simulink model "Integrate_and_fire_STDP"  (R2019b)
settings: Solver=VariableStepAuto  StartTime=0.0  StopTime=1  RelTol=1e-3
libraries: NeuroModelerLibrary x4
settings Model: Creator=Oleg  LastModifiedBy=Bakhshiev
settings DataIOCC: ReturnWorkspaceOutputs=off
settings DebuggingCC: ArithmeticOperatorsInVariantConditions=warning
settings SFSimCC: SimUseLocalCustomCode=off  CustomCodeUndefinedFunction=UseInterfaceOnly
settings RTWCC: RTWUseLocalCustomCode=off
settings CodeAppCC: StateflowObjectComments=on

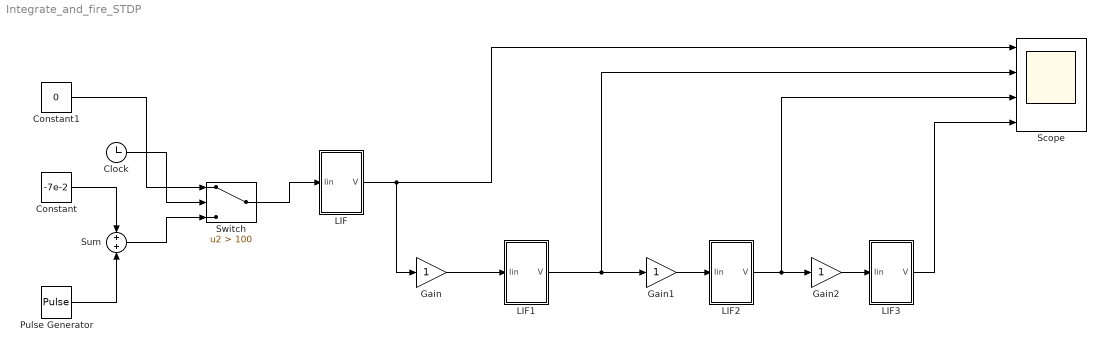
== system Integrate_and_fire_STDP ==
  Clock : Clock
  Constant : Constant  Value=-7e-2
  Constant1 : Constant  Value=0
  Gain : Gain
  Gain1 : Gain
  Gain2 : Gain
  LIF : Subsystem  mask{gL=3e-8, VL=-7e-2, C=1e-11, VT=-5e-2, Vreset=3e-2}
      mask prompts: gL "membraneConductivity (gL)"; VL "restingPotential (VL)"; C "capacity (C)"; VT "thresholdPotential (VT)"; Vreset "actionPotential (Vreset)"
  LIF1 : Subsystem  mask{gL=3e-8, VL=-7e-2, C=1e-11, VT=-5e-2, Vreset=3e-2}
      mask prompts: gL "membraneConductivity (gL)"; VL "restingPotential (VL)"; C "capacity (C)"; VT "thresholdPotential (VT)"; Vreset "actionPotential (Vreset)"
  LIF2 : Subsystem  mask{gL=3e-8, VL=-7e-2, C=1e-11, VT=-5e-2, Vreset=3e-2}
      mask prompts: gL "membraneConductivity (gL)"; VL "restingPotential (VL)"; C "capacity (C)"; VT "thresholdPotential (VT)"; Vreset "actionPotential (Vreset)"
  LIF3 : Subsystem  mask{gL=3e-8, VL=-7e-2, C=1e-11, VT=-5e-2, Vreset=3e-2}
      mask prompts: gL "membraneConductivity (gL)"; VL "restingPotential (VL)"; C "capacity (C)"; VT "thresholdPotential (VT)"; Vreset "actionPotential (Vreset)"
  Pulse Generator : DiscretePulseGenerator  PulseType=Time based  Amplitude=0.1  Period=0.1
  Scope : Scope  NumInputPorts=4
  Sum : Sum
  Switch : Switch  Criteria=u2 > Threshold  Threshold=100
  wires:
  LIF/1(V) -> Gain/1, Scope/1
  LIF1/1(V) -> Gain1/1, Scope/2
  Gain/1 -> LIF1/1(Iin)
  LIF2/1(V) -> Gain2/1, Scope/3
  LIF3/1(V) -> Scope/4
  Gain1/1 -> LIF2/1(Iin)
  Gain2/1 -> LIF3/1(Iin)
  Constant/1 -> Sum/1
  Pulse Generator/1 -> Sum/2
  Switch/1 -> LIF/1(Iin)
  Clock/1 -> Switch/2
  Constant1/1 -> Switch/1
  Sum/1 -> Switch/3

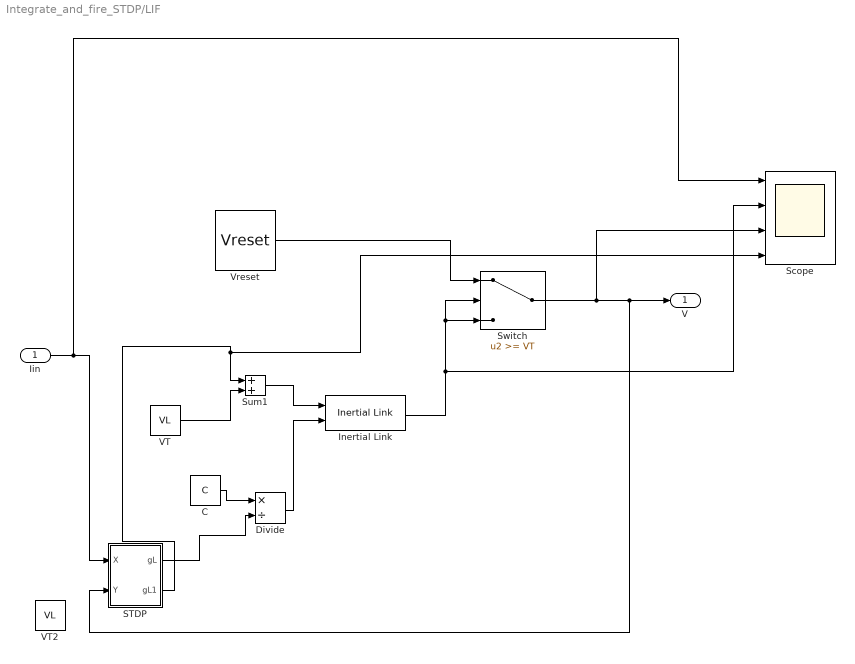
== system Integrate_and_fire_STDP/LIF ==
  Iin : Inport
  C : Constant  Value=C
  Divide : Product  Inputs=*/
  Inertial Link : NeuroModelerLibrary/Support/Inertial Link  SystemSampleTime=-1  Latency=0  AutoFrameSizeCalculation=off
  STDP : Subsystem
  Scope : Scope  NumInputPorts=4
  Sum1 : Sum
  Switch : Switch  Threshold=VT
  VT : Constant  Value=VL
  VT2 : Constant  Value=VL
  Vreset : Constant  Value=Vreset
  V : Outport
  wires:
  Inertial Link/1 -> Scope/2, Switch/2, Switch/3
  Sum1/1 -> Inertial Link/1
  Iin/1 -> STDP/1(X), Scope/1
  VT/1 -> Sum1/2
  C/1 -> Divide/1
  Divide/1 -> Inertial Link/2
  Vreset/1 -> Switch/1
  Switch/1 -> Scope/3, STDP/2(Y), V/1
  STDP/1(gL) -> Divide/2
  STDP/2(gL1) -> Scope/4, Sum1/1

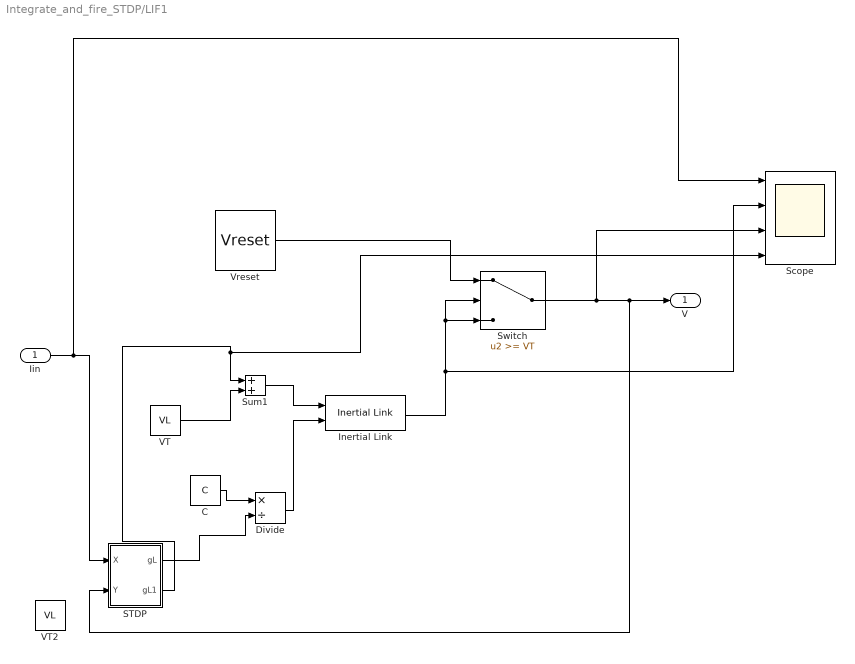
== system Integrate_and_fire_STDP/LIF1 ==
  Iin : Inport
  C : Constant  Value=C
  Divide : Product  Inputs=*/
  Inertial Link : NeuroModelerLibrary/Support/Inertial Link  SystemSampleTime=-1  Latency=0  AutoFrameSizeCalculation=off
  STDP : Subsystem
  Scope : Scope  NumInputPorts=4
  Sum1 : Sum
  Switch : Switch  Threshold=VT
  VT : Constant  Value=VL
  VT2 : Constant  Value=VL
  Vreset : Constant  Value=Vreset
  V : Outport
  wires:
  Inertial Link/1 -> Scope/2, Switch/2, Switch/3
  Sum1/1 -> Inertial Link/1
  Iin/1 -> STDP/1(X), Scope/1
  VT/1 -> Sum1/2
  C/1 -> Divide/1
  Divide/1 -> Inertial Link/2
  Vreset/1 -> Switch/1
  Switch/1 -> Scope/3, STDP/2(Y), V/1
  STDP/1(gL) -> Divide/2
  STDP/2(gL1) -> Scope/4, Sum1/1

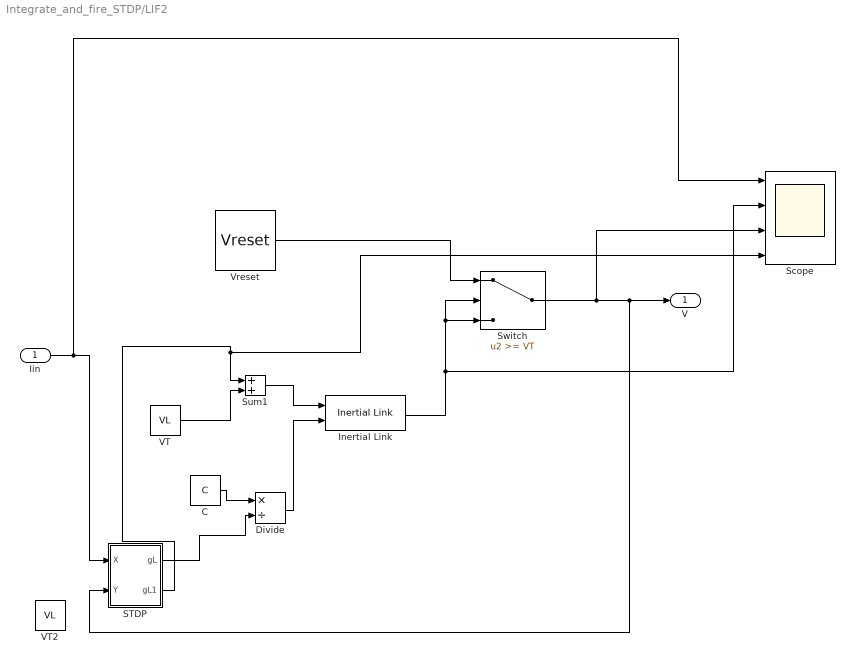
== system Integrate_and_fire_STDP/LIF2 ==
  Iin : Inport
  C : Constant  Value=C
  Divide : Product  Inputs=*/
  Inertial Link : NeuroModelerLibrary/Support/Inertial Link  SystemSampleTime=-1  Latency=0  AutoFrameSizeCalculation=off
  STDP : Subsystem
  Scope : Scope  NumInputPorts=4
  Sum1 : Sum
  Switch : Switch  Threshold=VT
  VT : Constant  Value=VL
  VT2 : Constant  Value=VL
  Vreset : Constant  Value=Vreset
  V : Outport
  wires:
  Inertial Link/1 -> Scope/2, Switch/2, Switch/3
  Sum1/1 -> Inertial Link/1
  Iin/1 -> STDP/1(X), Scope/1
  VT/1 -> Sum1/2
  C/1 -> Divide/1
  Divide/1 -> Inertial Link/2
  Vreset/1 -> Switch/1
  Switch/1 -> Scope/3, STDP/2(Y), V/1
  STDP/1(gL) -> Divide/2
  STDP/2(gL1) -> Scope/4, Sum1/1

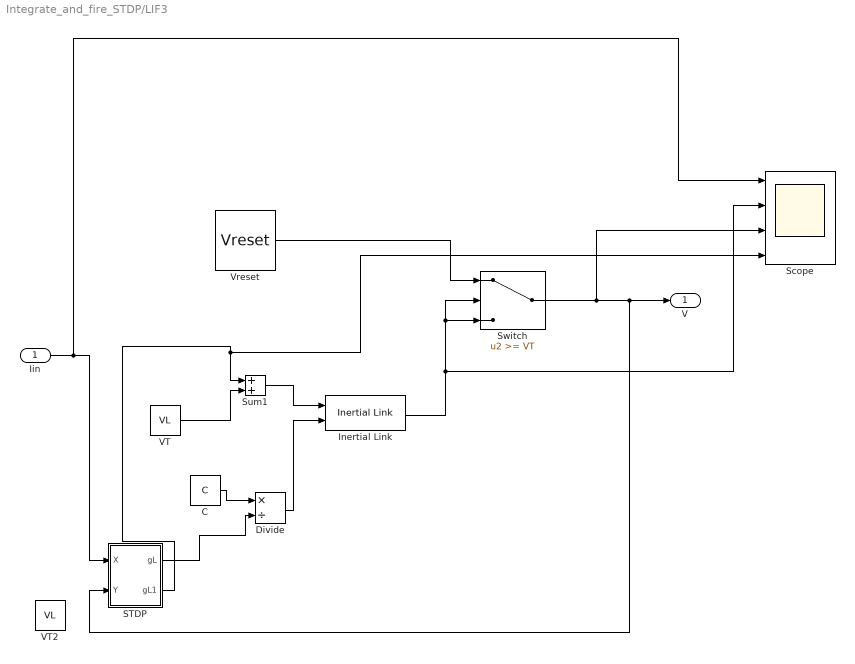
== system Integrate_and_fire_STDP/LIF3 ==
  Iin : Inport
  C : Constant  Value=C
  Divide : Product  Inputs=*/
  Inertial Link : NeuroModelerLibrary/Support/Inertial Link  SystemSampleTime=-1  Latency=0  AutoFrameSizeCalculation=off
  STDP : Subsystem
  Scope : Scope  NumInputPorts=4
  Sum1 : Sum
  Switch : Switch  Threshold=VT
  VT : Constant  Value=VL
  VT2 : Constant  Value=VL
  Vreset : Constant  Value=Vreset
  V : Outport
  wires:
  Inertial Link/1 -> Scope/2, Switch/2, Switch/3
  Sum1/1 -> Inertial Link/1
  Iin/1 -> STDP/1(X), Scope/1
  VT/1 -> Sum1/2
  C/1 -> Divide/1
  Divide/1 -> Inertial Link/2
  Vreset/1 -> Switch/1
  Switch/1 -> Scope/3, STDP/2(Y), V/1
  STDP/1(gL) -> Divide/2
  STDP/2(gL1) -> Scope/4, Sum1/1

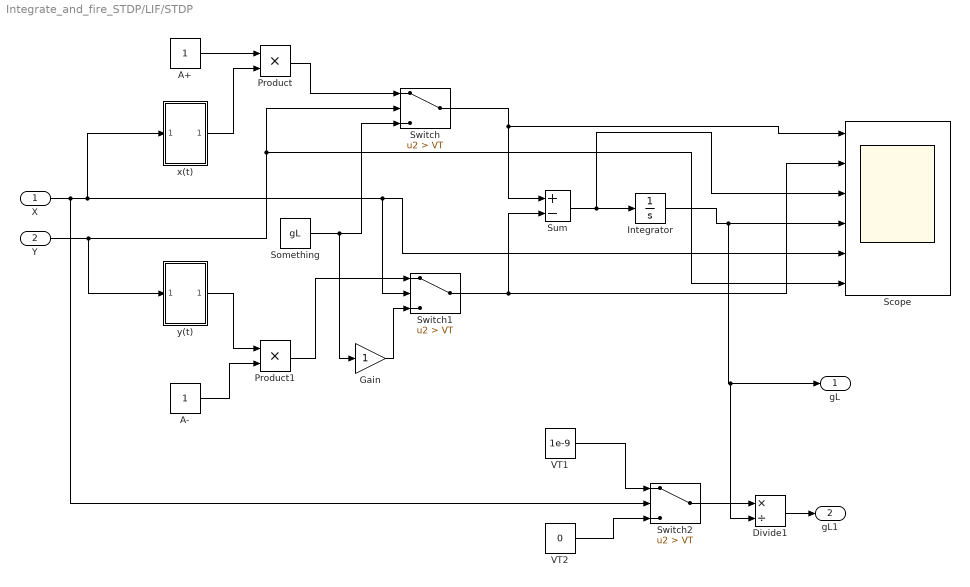
== system Integrate_and_fire_STDP/LIF/STDP ==
  X : Inport
  Y : Inport  Port=2
  A+ : Constant
  A- : Constant
  Divide1 : Product  Inputs=*/
  Gain : Gain
  Integrator : Integrator  InitialCondition=gL
  Product : Product
  Product1 : Product
  Scope : Scope  NumInputPorts=6
  Something : Constant  Value=gL
  Sum : Sum  Inputs=+-
  Switch : Switch  Criteria=u2 > Threshold  Threshold=VT
  Switch1 : Switch  Criteria=u2 > Threshold  Threshold=VT
  Switch2 : Switch  Criteria=u2 > Threshold  Threshold=VT
  VT1 : Constant  Value=1e-9
  VT2 : Constant  Value=0
  "x(t) " : Subsystem
  y(t) : Subsystem
  gL : Outport
  gL1 : Outport  Port=2
  wires:
  X/1 -> Switch2/2, "x(t) "/1(In1), Scope/5, Switch1/2
  Y/1 -> y(t)/1(In1), Scope/6, Switch/2
  A-/1 -> Product1/2
  Product1/1 -> Switch1/1
  Switch1/1 -> Scope/2, Sum/2
  A+/1 -> Product/1
  Product/1 -> Switch/1
  "x(t) "/1(Out1) -> Product/2
  Switch/1 -> Scope/1, Sum/1
  Something/1 -> Gain/1, Switch/3
  y(t)/1(Out1) -> Product1/1
  Sum/1 -> Integrator/1, Scope/3
  Gain/1 -> Switch1/3
  Integrator/1 -> Divide1/2, gL/1, Scope/4
  Divide1/1 -> gL1/1
  Switch2/1 -> Divide1/1
  VT1/1 -> Switch2/1
  VT2/1 -> Switch2/3

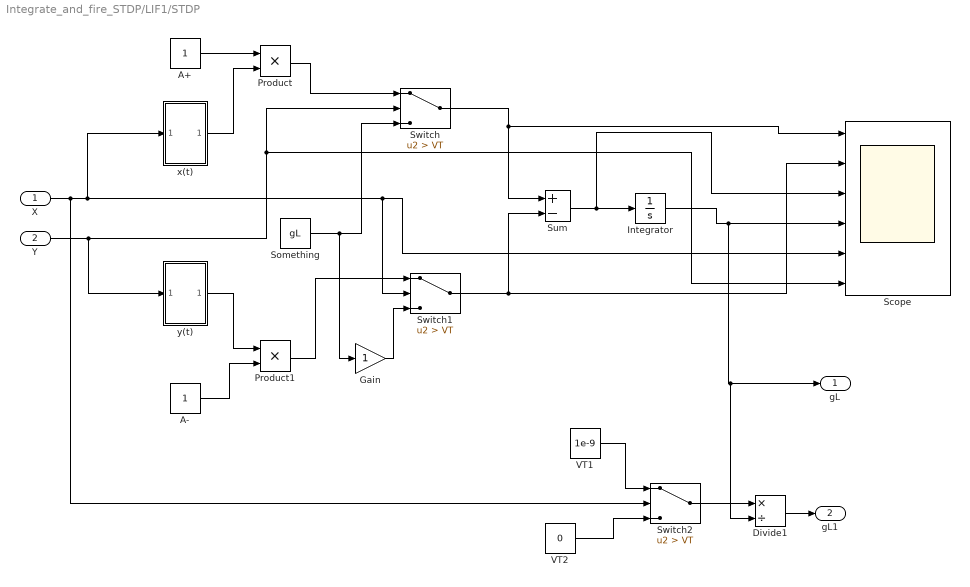
== system Integrate_and_fire_STDP/LIF1/STDP ==
  X : Inport
  Y : Inport  Port=2
  A+ : Constant
  A- : Constant
  Divide1 : Product  Inputs=*/
  Gain : Gain
  Integrator : Integrator  InitialCondition=gL
  Product : Product
  Product1 : Product
  Scope : Scope  NumInputPorts=6
  Something : Constant  Value=gL
  Sum : Sum  Inputs=+-
  Switch : Switch  Criteria=u2 > Threshold  Threshold=VT
  Switch1 : Switch  Criteria=u2 > Threshold  Threshold=VT
  Switch2 : Switch  Criteria=u2 > Threshold  Threshold=VT
  VT1 : Constant  Value=1e-9
  VT2 : Constant  Value=0
  "x(t) " : Subsystem
  y(t) : Subsystem
  gL : Outport
  gL1 : Outport  Port=2
  wires:
  X/1 -> Switch2/2, "x(t) "/1(In1), Scope/5, Switch1/2
  Y/1 -> y(t)/1(In1), Scope/6, Switch/2
  A-/1 -> Product1/2
  Product1/1 -> Switch1/1
  Switch1/1 -> Scope/2, Sum/2
  A+/1 -> Product/1
  Product/1 -> Switch/1
  "x(t) "/1(Out1) -> Product/2
  Switch/1 -> Scope/1, Sum/1
  Something/1 -> Gain/1, Switch/3
  y(t)/1(Out1) -> Product1/1
  Sum/1 -> Integrator/1, Scope/3
  Gain/1 -> Switch1/3
  Integrator/1 -> Divide1/2, gL/1, Scope/4
  Divide1/1 -> gL1/1
  Switch2/1 -> Divide1/1
  VT1/1 -> Switch2/1
  VT2/1 -> Switch2/3

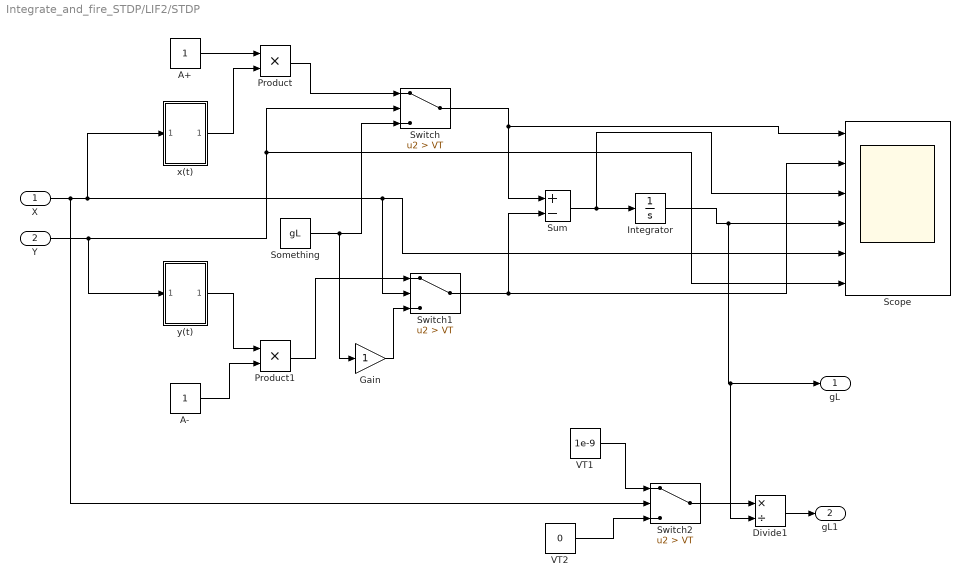
== system Integrate_and_fire_STDP/LIF2/STDP ==
  X : Inport
  Y : Inport  Port=2
  A+ : Constant
  A- : Constant
  Divide1 : Product  Inputs=*/
  Gain : Gain
  Integrator : Integrator  InitialCondition=gL
  Product : Product
  Product1 : Product
  Scope : Scope  NumInputPorts=6
  Something : Constant  Value=gL
  Sum : Sum  Inputs=+-
  Switch : Switch  Criteria=u2 > Threshold  Threshold=VT
  Switch1 : Switch  Criteria=u2 > Threshold  Threshold=VT
  Switch2 : Switch  Criteria=u2 > Threshold  Threshold=VT
  VT1 : Constant  Value=1e-9
  VT2 : Constant  Value=0
  "x(t) " : Subsystem
  y(t) : Subsystem
  gL : Outport
  gL1 : Outport  Port=2
  wires:
  X/1 -> Switch2/2, "x(t) "/1(In1), Scope/5, Switch1/2
  Y/1 -> y(t)/1(In1), Scope/6, Switch/2
  A-/1 -> Product1/2
  Product1/1 -> Switch1/1
  Switch1/1 -> Scope/2, Sum/2
  A+/1 -> Product/1
  Product/1 -> Switch/1
  "x(t) "/1(Out1) -> Product/2
  Switch/1 -> Scope/1, Sum/1
  Something/1 -> Gain/1, Switch/3
  y(t)/1(Out1) -> Product1/1
  Sum/1 -> Integrator/1, Scope/3
  Gain/1 -> Switch1/3
  Integrator/1 -> Divide1/2, gL/1, Scope/4
  Divide1/1 -> gL1/1
  Switch2/1 -> Divide1/1
  VT1/1 -> Switch2/1
  VT2/1 -> Switch2/3

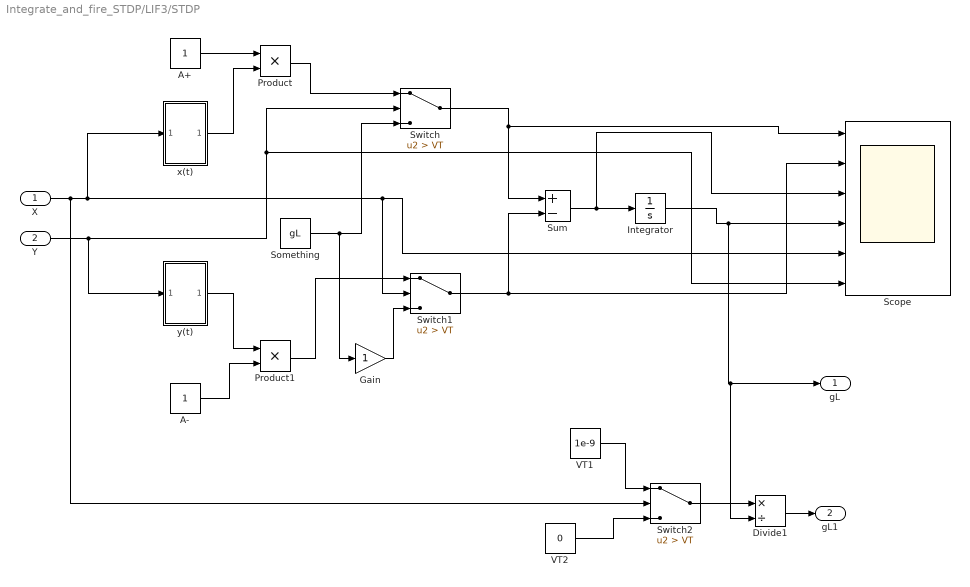
== system Integrate_and_fire_STDP/LIF3/STDP ==
  X : Inport
  Y : Inport  Port=2
  A+ : Constant
  A- : Constant
  Divide1 : Product  Inputs=*/
  Gain : Gain
  Integrator : Integrator  InitialCondition=gL
  Product : Product
  Product1 : Product
  Scope : Scope  NumInputPorts=6
  Something : Constant  Value=gL
  Sum : Sum  Inputs=+-
  Switch : Switch  Criteria=u2 > Threshold  Threshold=VT
  Switch1 : Switch  Criteria=u2 > Threshold  Threshold=VT
  Switch2 : Switch  Criteria=u2 > Threshold  Threshold=VT
  VT1 : Constant  Value=1e-9
  VT2 : Constant  Value=0
  "x(t) " : Subsystem
  y(t) : Subsystem
  gL : Outport
  gL1 : Outport  Port=2
  wires:
  X/1 -> Switch2/2, "x(t) "/1(In1), Scope/5, Switch1/2
  Y/1 -> y(t)/1(In1), Scope/6, Switch/2
  A-/1 -> Product1/2
  Product1/1 -> Switch1/1
  Switch1/1 -> Scope/2, Sum/2
  A+/1 -> Product/1
  Product/1 -> Switch/1
  "x(t) "/1(Out1) -> Product/2
  Switch/1 -> Scope/1, Sum/1
  Something/1 -> Gain/1, Switch/3
  y(t)/1(Out1) -> Product1/1
  Sum/1 -> Integrator/1, Scope/3
  Gain/1 -> Switch1/3
  Integrator/1 -> Divide1/2, gL/1, Scope/4
  Divide1/1 -> gL1/1
  Switch2/1 -> Divide1/1
  VT1/1 -> Switch2/1
  VT2/1 -> Switch2/3

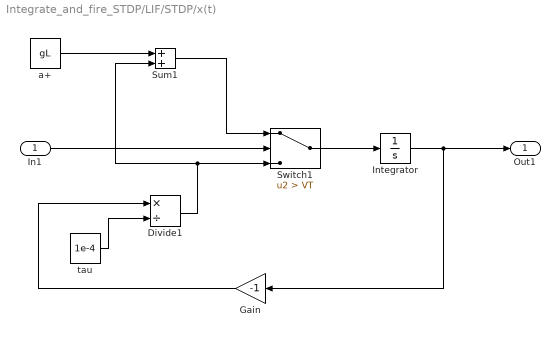
== system Integrate_and_fire_STDP/LIF/STDP/x(t)  ==
  In1 : Inport
  Divide1 : Product  Inputs=*/
  Gain : Gain  Gain=-1
  Integrator : Integrator
  Sum1 : Sum
  Switch1 : Switch  Criteria=u2 > Threshold  Threshold=VT
  a+ : Constant  Value=gL
  tau : Constant  Value=1e-4
  Out1 : Outport
  wires:
  Integrator/1 -> Gain/1, Out1/1
  In1/1 -> Switch1/2
  a+/1 -> Sum1/1
  Gain/1 -> Divide1/1
  tau/1 -> Divide1/2
  Divide1/1 -> Sum1/2, Switch1/3
  Sum1/1 -> Switch1/1
  Switch1/1 -> Integrator/1

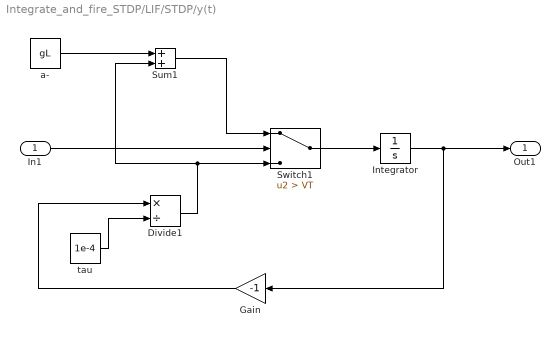
== system Integrate_and_fire_STDP/LIF/STDP/y(t) ==
  In1 : Inport
  Divide1 : Product  Inputs=*/
  Gain : Gain  Gain=-1
  Integrator : Integrator
  Sum1 : Sum
  Switch1 : Switch  Criteria=u2 > Threshold  Threshold=VT
  a- : Constant  Value=gL
  tau : Constant  Value=1e-4
  Out1 : Outport
  wires:
  Switch1/1 -> Integrator/1
  Sum1/1 -> Switch1/1
  Divide1/1 -> Switch1/3, Sum1/2
  tau/1 -> Divide1/2
  Gain/1 -> Divide1/1
  a-/1 -> Sum1/1
  In1/1 -> Switch1/2
  Integrator/1 -> Out1/1, Gain/1

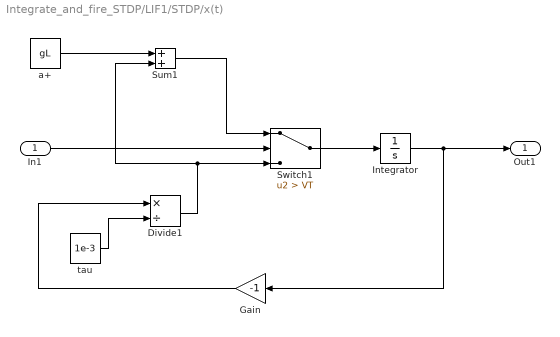
== system Integrate_and_fire_STDP/LIF1/STDP/x(t)  ==
  In1 : Inport
  Divide1 : Product  Inputs=*/
  Gain : Gain  Gain=-1
  Integrator : Integrator
  Sum1 : Sum
  Switch1 : Switch  Criteria=u2 > Threshold  Threshold=VT
  a+ : Constant  Value=gL
  tau : Constant  Value=1e-3
  Out1 : Outport
  wires:
  Integrator/1 -> Gain/1, Out1/1
  In1/1 -> Switch1/2
  a+/1 -> Sum1/1
  Gain/1 -> Divide1/1
  tau/1 -> Divide1/2
  Divide1/1 -> Sum1/2, Switch1/3
  Sum1/1 -> Switch1/1
  Switch1/1 -> Integrator/1

== system Integrate_and_fire_STDP/LIF1/STDP/y(t) ==
  In1 : Inport
  Divide1 : Product  Inputs=*/
  Gain : Gain  Gain=-1
  Integrator : Integrator
  Sum1 : Sum
  Switch1 : Switch  Criteria=u2 > Threshold  Threshold=VT
  a- : Constant  Value=gL
  tau : Constant  Value=1e-3
  Out1 : Outport
  wires:
  Switch1/1 -> Integrator/1
  Sum1/1 -> Switch1/1
  Divide1/1 -> Switch1/3, Sum1/2
  tau/1 -> Divide1/2
  Gain/1 -> Divide1/1
  a-/1 -> Sum1/1
  In1/1 -> Switch1/2
  Integrator/1 -> Out1/1, Gain/1

== system Integrate_and_fire_STDP/LIF2/STDP/x(t)  ==
  In1 : Inport
  Divide1 : Product  Inputs=*/
  Gain : Gain  Gain=-1
  Integrator : Integrator
  Sum1 : Sum
  Switch1 : Switch  Criteria=u2 > Threshold  Threshold=VT
  a+ : Constant  Value=gL
  tau : Constant  Value=1e-3
  Out1 : Outport
  wires:
  Integrator/1 -> Gain/1, Out1/1
  In1/1 -> Switch1/2
  a+/1 -> Sum1/1
  Gain/1 -> Divide1/1
  tau/1 -> Divide1/2
  Divide1/1 -> Sum1/2, Switch1/3
  Sum1/1 -> Switch1/1
  Switch1/1 -> Integrator/1

== system Integrate_and_fire_STDP/LIF2/STDP/y(t) ==
  In1 : Inport
  Divide1 : Product  Inputs=*/
  Gain : Gain  Gain=-1
  Integrator : Integrator
  Sum1 : Sum
  Switch1 : Switch  Criteria=u2 > Threshold  Threshold=VT
  a- : Constant  Value=gL
  tau : Constant  Value=1e-3
  Out1 : Outport
  wires:
  Switch1/1 -> Integrator/1
  Sum1/1 -> Switch1/1
  Divide1/1 -> Switch1/3, Sum1/2
  tau/1 -> Divide1/2
  Gain/1 -> Divide1/1
  a-/1 -> Sum1/1
  In1/1 -> Switch1/2
  Integrator/1 -> Out1/1, Gain/1

== system Integrate_and_fire_STDP/LIF3/STDP/x(t)  ==
  In1 : Inport
  Divide1 : Product  Inputs=*/
  Gain : Gain  Gain=-1
  Integrator : Integrator
  Sum1 : Sum
  Switch1 : Switch  Criteria=u2 > Threshold  Threshold=VT
  a+ : Constant  Value=gL
  tau : Constant  Value=1e-3
  Out1 : Outport
  wires:
  Integrator/1 -> Gain/1, Out1/1
  In1/1 -> Switch1/2
  a+/1 -> Sum1/1
  Gain/1 -> Divide1/1
  tau/1 -> Divide1/2
  Divide1/1 -> Sum1/2, Switch1/3
  Sum1/1 -> Switch1/1
  Switch1/1 -> Integrator/1

== system Integrate_and_fire_STDP/LIF3/STDP/y(t) ==
  In1 : Inport
  Divide1 : Product  Inputs=*/
  Gain : Gain  Gain=-1
  Integrator : Integrator
  Sum1 : Sum
  Switch1 : Switch  Criteria=u2 > Threshold  Threshold=VT
  a- : Constant  Value=gL
  tau : Constant  Value=1e-3
  Out1 : Outport
  wires:
  Switch1/1 -> Integrator/1
  Sum1/1 -> Switch1/1
  Divide1/1 -> Switch1/3, Sum1/2
  tau/1 -> Divide1/2
  Gain/1 -> Divide1/1
  a-/1 -> Sum1/1
  In1/1 -> Switch1/2
  Integrator/1 -> Out1/1, Gain/1
